simulink library "thermochemical"  (R2017b)
settings: Solver=VariableStepAuto  StartTime=0.0  StopTime=10.0  RelTol=1e-3
values from neighbouring files (symbols this model uses):
  c = conversion_factors()    [blk_clausius_clapeyron.m]    (also in blk_clausius_clapeyron_no_popup.m; blk_cold_room_closed_dry_air.m; blk_reactor_BaCl2_NH3_no_walls.m; blk_reactor_BaCl2_NH3_no_walls_state_space.m)
  cp = metal.cp    [blk_wall_simple.m]    (also in get_metal_properties.m = 390)
  fluid = get_param(blk,'fluid')    [blk_thermodynamic_properties_nonsaturated.m]    (also in blk_thermodynamic_properties_nonsaturated_interpreted.m; blk_thermodynamic_properties_saturated.m; blk_thermodynamic_properties_saturated_interpreted.m; blk_thermodynamic_properties_saturated_mix.m)
  gas = get_material_properties(x.gasName)    [blk_reactor_BaCl2_NH3_cylindrical_no_walls_fun1.m]
  h = get_param(gcb,'ObjectParameters')    [get_param_eval.m]
  rho = metal.rho    [blk_wall_simple.m]    (also in get_metal_properties.m = 8940)
  s = solve(eq,dx,'ReturnConditions',true)    [LMTD_inv.m]    (also in blk_wall_simple.m = get_param_eval(blk,'s'))
  u_gas_at_T_ref = -R * T_ref    [blk_reactor_BaCl2_NH3_no_walls.m]    (also in blk_reactor_BaCl2_NH3_no_walls_state_space.m)
undefined symbols (not defined in the file or in its folder): b_motor, BaCl2, beta, CoolProp, cP_binder, cP_gas, cP_s0, cv, dh_r_0, ENG, heat_exchanger_epsilonNTU_inv_simulink, heat_exchanger_epsilonNTU_simulink, J_motor, K_cin, kappa, Km_motor, La_motor, lookup2D_BreakPoint2, M_binder, N_binder, N_gas_free_volume_init, N_salt, NH3, nh3_v3, nu, P, phase, PID_D_motor, PID_I_motor, PID_P_motor, Ra_motor, Reactor_phase, T, T1, T2, T_init, Tr_init, Tr_ref, U_binder_at_Tr_ref, U_salt_at_X0_Tr_ref, Ur_init, V_void, Valve_regime, Vmax_motor, w_init_motor, X_init
libraries: thermochemical x247, simulink x54, dspsigops x3
(part 10 of 12)

== system thermochemical/Reactors/Reactor, BaCl2//NH3, with algebraic loops, real gas in void volume, ideal gas in salt/Reactor, BaCl2//NH3, no walls, with algebraic loops, real gas in void volume, ideal gas in salt/Reactor (no walls)/Reactor's temperature and pressure ==
  In2 : Inport
  In1 : Inport  Port=2
  "Reaction kinetic, differential equation" : Subsystem
  Reactor's energy balance : Subsystem
  Out3 : Outport
  Out1 : Outport  Port=2
  Out2 : Outport  Port=3
  Out4 : Outport  Port=4
  wires:
  "Reaction kinetic, differential equation"/1(Out1) -> Out2/1  "Reactor phase"
  Reactor's energy balance/2(Out2) -> Out1/1, "Reaction kinetic, differential equation"/2(In2)  "P_reactor (bar)"
  In2/1 -> Reactor's energy balance/2(In2)  "N_gas_reactor (mol)"
  Reactor's energy balance/1(Out1) -> Out3/1, "Reaction kinetic, differential equation"/1(In1)  "T_reactor (K)"
  "Reaction kinetic, differential equation"/2(Out2) -> Reactor's energy balance/3(In3), Out4/1  "X (0..1)"
  In1/1 -> Reactor's energy balance/1(In1)  "U_reactor (J)"

== system thermochemical/Reactors/Reactor, BaCl2//NH3, with algebraic loops, real gas in void volume, real gas in salt/Reactor, BaCl2//NH3, no walls, with algebraic loops, real gas in void volume, real gas in salt/Reactor (no walls)/Reactor's internal energy differential equation ==
  note: Reactor - Internal energy's
      | differential equation
  In1 : Inport
  In2 : Inport  Port=2
  In5 : Inport  Port=3
  In3 : Inport  Port=4
  1 : Constant  Value=X_init
  2 : Constant  Value=N_gas_free_volume_init
  3 : Constant  Value=Tr_init
  Integrator6 : Integrator  InitialConditionSource=external  InitialCondition=Ur_init
  Product4 : Product
  Reactor's internal energy equation : thermochemical/Reactors/Reactor's internal energy equation  Tr_ref=T_ref  N_salt=N_salt  cP_s0=cP_s0  U_salt_at_X0_Tr_ref=U_salt_at_X0_T_ref  N_binder=N_binder  M_binder=M_binder  cP_binder=cP_binder  U_binder_at_Tr_ref=U_binder_at_T_ref  V_void=V_void  gas_model_void_volume=Real gas model  gas_model_salt=Real gas model  is_ideal_gas_in_void_volume=-1  is_ideal_gas_in_salt=-1  fluid=fluid  cP_gas=cP_gas  u_gas_at_Tr_ref=u_gas_at_T_ref  nu=nu  dh_r=dh_r_0  R=8.314472
      settings: SourceProductName=@ Thermochemical
  Relay : Relay  OnSwitchValue=dn_dead_zone  OffSwitchValue=-dn_dead_zone  OffOutputValue=-1
  Sum19 : Sum  Inputs=++|
  Switch1 : Switch
  Out1 : Outport
  wires:
  In3/1 -> Relay/1, Product4/2  "dn_gas (mol/sec) > 0: gas in   < 0: gas out"
  In5/1 -> Switch1/3  "enthalpy out (J/mol)"
  In1/1 -> Sum19/1  "q out → in (W)"
  Sum19/1 -> Integrator6/1  "dUr"
  Integrator6/1 -> Out1/1  "U_reactor (J)"
  In2/1 -> Switch1/1  "enthalpy in (J/mol)"
  Switch1/1 -> Product4/1  "h_gas(Tgas)"
  Product4/1 -> Sum19/2  "dn_gas * h_gas"
  Reactor's internal energy equation/1 -> Integrator6/2
  1/1 -> Reactor's internal energy equation/1
  3/1 -> Reactor's internal energy equation/3
  2/1 -> Reactor's internal energy equation/2
  Relay/1 -> Switch1/2

== system thermochemical/Reactors/Reactor, BaCl2//NH3, with algebraic loops, real gas in void volume, real gas in salt/Reactor, BaCl2//NH3, no walls, with algebraic loops, real gas in void volume, real gas in salt/Reactor (no walls)/Reactor's temperature and pressure ==
  In2 : Inport
  In1 : Inport  Port=2
  "Reaction kinetic, differential equation" : Subsystem
  Reactor's energy balance : Subsystem
  Out3 : Outport
  Out1 : Outport  Port=2
  Out2 : Outport  Port=3
  Out4 : Outport  Port=4
  wires:
  In1/1 -> Reactor's energy balance/1(In1)  "U_reactor (J)"
  "Reaction kinetic, differential equation"/2(Out2) -> Out4/1, Reactor's energy balance/3(In3)  "X (0..1)"
  Reactor's energy balance/1(Out1) -> "Reaction kinetic, differential equation"/1(In1), Out3/1  "T_reactor (K)"
  In2/1 -> Reactor's energy balance/2(In2)  "N_gas_reactor (mol)"
  Reactor's energy balance/2(Out2) -> "Reaction kinetic, differential equation"/2(In2), Out1/1  "P_reactor (bar)"
  "Reaction kinetic, differential equation"/1(Out1) -> Out2/1  "Reactor phase"

== system thermochemical/Valves/Valve, liquid, IEC 60534-2-1:2012/Flow computation for incompressible fluids, IEC 60534-2-1:2012/dP sizing computation/dP chocked computation ==
  P upstream (bar)1 : Inport
  P upstream (bar)2 : Inport  Port=2
  P upstream (bar)3 : Inport  Port=3
  P upstream (bar)4 : Inport  Port=4
  Display1 : Display
  Display2 : Display
  Display3 : Display
  "Liquid critical pressure ratio factor, FF" : Subsystem
  Math Function : Math  Operator=square  SaturateOnIntegerOverflow=on
  Prod1 : Product  Inputs=**
  Prod2 : Product  Inputs=**
  Sum2 : Sum  Inputs=+-
  dP chocked (bar) : Outport
  wires:
  Sum2/1 -> Prod2/1
  Prod2/1 -> dP chocked (bar)/1  "dP chocked (bar)"
  Prod1/1 -> Display1/1, Sum2/2
  Math Function/1 -> Prod2/2
  P upstream (bar)4/1 -> Math Function/1  "FF factor"
  "Liquid critical pressure ratio factor, FF"/1(FF) -> Prod1/2, Display3/1
  P upstream (bar)3/1 -> "Liquid critical pressure ratio factor, FF"/2(P upstream (bar)1)  "Pc: absolute thermodynamic  critical pressure (bar)"
  P upstream (bar)1/1 -> Sum2/1  "P upstream (bar)"
  P upstream (bar)2/1 -> Prod1/1, Display2/1, "Liquid critical pressure ratio factor, FF"/1(P upstream (bar)2)  "Pv: absolute vapor pressure  of liquid at T upstream (bar)"

== system thermochemical/Walls/Wall, tube with//without fins/Subsystem1/Subsystem2/Subsystem1 ==
  In1 : Inport
  In2 : Inport  Port=2
  In3 : Inport  Port=3
  Gain1 : Gain  Gain=pi/4
  Gain2 : Gain  Gain=2
  Gain4 : Gain  Gain=1e-3
  Gain5 : Gain  Gain=1e-3
  Math Function : Math  Operator=square  SaturateOnIntegerOverflow=on
  Math Function1 : Math  Operator=square  SaturateOnIntegerOverflow=on
  Product2 : Product
  Sum1 : Sum  Inputs=+-
  Sum2 : Sum  Inputs=+-
  Inner area (m2) : Outport
  wires:
  Gain1/1 -> Product2/1
  Product2/1 -> Inner area (m2)/1  "Bare tube volume (m3)"
  In3/1 -> Product2/2  "L_m"
  In1/1 -> Gain4/1  "OD_mm"
  In2/1 -> Gain5/1  "e_mm"
  Sum1/1 -> Math Function1/1
  Math Function/1 -> Sum2/1
  Math Function1/1 -> Sum2/2
  Sum2/1 -> Gain1/1
  Gain4/1 -> Sum1/1, Math Function/1  "OD_m"
  Gain5/1 -> Gain2/1  "e_m"
  Gain2/1 -> Sum1/2

== system thermochemical/Walls/Wall, tube with//without fins/Subsystem1/Subsystem2/Subsystem2 ==
  In1 : Inport
  In2 : Inport  Port=2
  In4 : Inport  Port=3
  Gain1 : Gain  Gain=pi/4
  Gain3 : Gain  Gain=1e-3
  Gain4 : Gain  Gain=1e-3
  Gain5 : Gain  Gain=1e-3
  Math Function : Math  Operator=square  SaturateOnIntegerOverflow=on
  Math Function1 : Math  Operator=square  SaturateOnIntegerOverflow=on
  Product : Product
  Sum2 : Sum  Inputs=+-
  Sum3 : Sum
  Inner area (m2) : Outport
  wires:
  Product/1 -> Inner area (m2)/1  "Volume of  individual fin (m3)"
  Gain3/1 -> Product/2  "thickness_fin_m"
  In2/1 -> Gain3/1  "thickness_fin_mm"
  Sum3/1 -> Math Function/1
  Gain1/1 -> Product/1  "Individual one-side  area of fin (m2)"
  In1/1 -> Gain5/1  "OD_mm"
  In4/1 -> Gain4/1  "height_fin_mm"
  Math Function/1 -> Sum2/1
  Math Function1/1 -> Sum2/2
  Sum2/1 -> Gain1/1
  Gain4/1 -> Sum3/1  "height_fin_m"
  Gain5/1 -> Sum3/2, Math Function1/1  "OD_m"

== system thermochemical/Walls/Wall, tube with//without fins, with internal heat production/Subsystem1/Subsystem2/Subsystem1 ==
  In1 : Inport
  In2 : Inport  Port=2
  In3 : Inport  Port=3
  Gain1 : Gain  Gain=pi/4
  Gain2 : Gain  Gain=2
  Gain4 : Gain  Gain=1e-3
  Gain5 : Gain  Gain=1e-3
  Math Function : Math  Operator=square  SaturateOnIntegerOverflow=on
  Math Function1 : Math  Operator=square  SaturateOnIntegerOverflow=on
  Product2 : Product
  Sum1 : Sum  Inputs=+-
  Sum2 : Sum  Inputs=+-
  Inner area (m2) : Outport
  wires:
  Gain5/1 -> Gain2/1  "e_m"
  Gain4/1 -> Math Function/1, Sum1/1  "OD_m"
  Sum2/1 -> Gain1/1
  Math Function1/1 -> Sum2/2
  Math Function/1 -> Sum2/1
  Sum1/1 -> Math Function1/1
  In2/1 -> Gain5/1  "e_mm"
  In1/1 -> Gain4/1  "OD_mm"
  In3/1 -> Product2/2  "L_m"
  Product2/1 -> Inner area (m2)/1  "Bare tube volume (m3)"
  Gain1/1 -> Product2/1
  Gain2/1 -> Sum1/2

== system thermochemical/Walls/Wall, tube with//without fins, with internal heat production/Subsystem1/Subsystem2/Subsystem2 ==
  In1 : Inport
  In2 : Inport  Port=2
  In4 : Inport  Port=3
  Gain1 : Gain  Gain=pi/4
  Gain3 : Gain  Gain=1e-3
  Gain4 : Gain  Gain=1e-3
  Gain5 : Gain  Gain=1e-3
  Math Function : Math  Operator=square  SaturateOnIntegerOverflow=on
  Math Function1 : Math  Operator=square  SaturateOnIntegerOverflow=on
  Product : Product
  Sum2 : Sum  Inputs=+-
  Sum3 : Sum
  Inner area (m2) : Outport
  wires:
  Gain5/1 -> Math Function1/1, Sum3/2  "OD_m"
  Gain4/1 -> Sum3/1  "height_fin_m"
  Sum2/1 -> Gain1/1
  Math Function1/1 -> Sum2/2
  Math Function/1 -> Sum2/1
  In4/1 -> Gain4/1  "height_fin_mm"
  In1/1 -> Gain5/1  "OD_mm"
  Gain1/1 -> Product/1  "Individual one-side  area of fin (m2)"
  Sum3/1 -> Math Function/1
  In2/1 -> Gain3/1  "thickness_fin_mm"
  Gain3/1 -> Product/2  "thickness_fin_m"
  Product/1 -> Inner area (m2)/1  "Volume of  individual fin (m3)"

== system thermochemical/Reactors/Reactor, BaCl2//NH3, state-space form, [Tr, Ng, X] as state variables, no algebraic loops, ideal gas in void volume, ideal gas in salt/Reactor, BaCl2//NH3, no walls, state-space form, [Tr, Ng, X] as state variables, no algebraic loops, ideal gas in void volume/Reactor, no walls, state space form/Reactor output function/Reactor phase ==
  In1 : Inport
  3 : Constant  Value=P_dead_zone
  Abs : Abs
  Enumerated Constant : simulink/Sources/Enumerated Constant  OutDataTypeStr=Enum: Reactor_phase  Value=Reactor_phase.Synthesis  SampleTime=inf
      settings: SourceProductName=Simulink
  Enumerated Constant1 : simulink/Sources/Enumerated Constant  OutDataTypeStr=Enum: Reactor_phase  Value=Reactor_phase.Desorption  SampleTime=inf
      settings: SourceProductName=Simulink
  Enumerated Constant2 : simulink/Sources/Enumerated Constant  OutDataTypeStr=Enum: Reactor_phase  Value=Reactor_phase.No_reaction  SampleTime=inf
      settings: SourceProductName=Simulink
  Relay : Relay  OnSwitchValue=P_dead_zone  OffSwitchValue=-P_dead_zone  OffOutputValue=-1
  Sign : Signum
  Sum17 : Sum  Inputs=|+-
  Switch1 : Switch  Criteria=u2 > Threshold
  Switch2 : Switch  Criteria=u2 > Threshold
  Out1 : Outport
  wires:
  Switch2/1 -> Out1/1  "Reactor phase"
  Enumerated Constant/1 -> Switch1/1  "Synthesis"
  Enumerated Constant1/1 -> Switch1/3  "Decomposition (desporption)"
  Switch1/1 -> Switch2/1
  Enumerated Constant2/1 -> Switch2/3  "No reaction"
  In1/1 -> Relay/1, Abs/1  "ΔP"
  Relay/1 -> Switch1/2
  Sum17/1 -> Sign/1
  Abs/1 -> Sum17/1
  Sign/1 -> Switch2/2
  3/1 -> Sum17/2

== system thermochemical/Reactors/Reactor, BaCl2//NH3, state-space form, [Tr, Ng, X] as state variables, no algebraic loops, ideal gas in void volume, ideal gas in salt/Reactor, BaCl2//NH3, no walls, state-space form, [Tr, Ng, X] as state variables, no algebraic loops, ideal gas in void volume/Reactor, no walls, state space form/Reactor state-space functions/f1 ==
  In6 : Inport
  In1 : Inport  Port=2
  Demux : Demux  Outputs=3
  Demux1 : Demux  Outputs=3
  Enthalpy of ideal gas : thermochemical/Thermodynamic fluid properties/Enthalpy of ideal gas  T_ref=T_ref  cP_gas=cP_gas  h_gas_at_T_ref="u_gas_at_T_ref  + R * T_ref"
      settings: SourceProductName=@ Thermochemical
  Enthalpy of reaction per mole of gas : Constant  Value=dh_r_0  VectorParams1D=off
  Gain2 : Gain  Gain=nu*N_salt
  Internal energy of ideal gas : thermochemical/Thermodynamic fluid properties/Internal energy of ideal gas  T_ref=T_ref  Cv_gas=cV_gas  u_gas_at_T_ref=u_gas_at_T_ref
      settings: SourceProductName=@ Thermochemical
  Product : Product  Inputs=/*
  Product1 : Product
  Product4 : Product
  Reactor's internal energy differential equation : thermochemical/Reactors/Reactor, BaCl2//NH3, state-space form, [Ur, Ng, X] as state variables, no algebraic loops, ideal gas in void volume, ideal gas in salt/Reactor, BaCl2//NH3, no walls, state-space form, [Ur, Ng, X] as state variables, no algebraic loops, ideal gas in void volume, ideal gas in salt/Reactor, no walls, state space form/Reactor state-space functions/f1/Reactor's internal energy differential equation
      settings: SourceProductName=@ Thermochemical
  Sum : Sum  Inputs=-+
  Sum3 : Sum  Inputs=--+
  Sum4 : Sum  Inputs=+-
  denominator : Subsystem
  f3 : Subsystem
  Out2 : Outport
  wires:
  Enthalpy of reaction per mole of gas/1 -> Sum/1  "(J/mol of gas)"
  Sum/1 -> Sum4/1  "(J/mol gas)"
  Enthalpy of ideal gas/1 -> Sum/2, Reactor's internal energy differential equation/3  "h gas"
  Product1/1 -> Sum3/2  "(J/sec)"
  Product4/1 -> Sum3/1  "(J/sec)"
  Reactor's internal energy differential equation/1 -> Sum3/3  "(J/sec)"
  Sum3/1 -> Product/2  "(J/sec)"
  f3/1(Out2) -> Product4/1  "(1/sec)"
  Gain2/1 -> Product4/2  "(J)"
  Sum4/1 -> Gain2/1
  Internal energy of ideal gas/1 -> Product1/1, Sum4/2  "J/mol"
  denominator/1(Out2) -> Product/1  "J/K"
  Demux/1 -> f3/1(In6), Enthalpy of ideal gas/1, Internal energy of ideal gas/1, denominator/1(In6)  "x(1) = T (K)"
  Demux1/3 -> Reactor's internal energy differential equation/1  "u(3) = Q out→in (W)"
  In1/1 -> Demux1/1  "U"
  Demux1/1 -> Reactor's internal energy differential equation/4, Product1/2  "u(1) = dn/dt gas (mol/sec), > 0: gas in, < 0: gas out"
  Demux1/2 -> Reactor's internal energy differential equation/2  "u(2) = h gas in (J/mol)"
  Demux/3 -> f3/3(In2), denominator/3(In4)  "x(3) = X (0..1)"
  Demux/2 -> f3/2(In1), denominator/2(In3)  "x(2) = Ngas,total (mol)"
  Product/1 -> Out2/1  "dT/dt (K/sec)"
  In6/1 -> Demux/1  "X"

== system thermochemical/Reactors/Reactor, BaCl2//NH3, state-space form, [Tr, Ng, X] as state variables, no algebraic loops, ideal gas in void volume, ideal gas in salt/Reactor, BaCl2//NH3, no walls, state-space form, [Tr, Ng, X] as state variables, no algebraic loops, ideal gas in void volume/Reactor, no walls, state space form/Reactor state-space functions/f2 ==
  In6 : Inport
  In2 : Inport  Port=2
  Demux : Demux  Outputs=3
  Demux2 : Demux  Outputs=3
  Gain : Gain
  Terminator{,1..2,5..6} (5 alike) : Terminator
  Out2 : Outport
  wires:
  Demux/1 -> Terminator/1  "x(1) = T (K)"
  In6/1 -> Demux/1  "X"
  Gain/1 -> Out2/1  "dNgas,total/dt (mol/sec)"
  Demux/2 -> Terminator1/1  "x(2) = Ngas,total (mol)"
  Demux/3 -> Terminator2/1  "x(3) = X (0..1)"
  Demux2/3 -> Terminator5/1  "u(3) = Q out→in (W)"
  Demux2/1 -> Gain/1  "u(1) = dn/dt gas (mol/sec), > 0: gas in, < 0: gas out"
  Demux2/2 -> Terminator6/1  "u(2) = h gas in (J/mol)"
  In2/1 -> Demux2/1  "U"

== system thermochemical/Reactors/Reactor, BaCl2//NH3, state-space form, [Tr, Ng, X] as state variables, no algebraic loops, ideal gas in void volume, ideal gas in salt/Reactor, BaCl2//NH3, no walls, state-space form, [Tr, Ng, X] as state variables, no algebraic loops, ideal gas in void volume/Reactor, no walls, state space form/Reactor state-space functions/f3 ==
  In6 : Inport
  In2 : Inport  Port=2
  Demux : Demux  Outputs=3
  Demux2 : Demux  Outputs=3
  Terminator1 : Terminator
  Terminator5 : Terminator
  Terminator6 : Terminator
  f3 : Subsystem
  Out2 : Outport
  wires:
  In6/1 -> Demux/1  "X"
  Demux/3 -> f3/3(In2)  "x(3) = X (0..1)"
  Demux/2 -> f3/2(In1)  "x(2) = Ngas,total (mol)"
  Demux/1 -> f3/1(In6)  "x(1) = T (K)"
  f3/1(Out2) -> Out2/1  "dX/dt (1/sec)"
  In2/1 -> Demux2/1  "U"
  Demux2/1 -> Terminator1/1  "u(1) = dn/dt gas (mol/sec), > 0: gas in, < 0: gas out"
  Demux2/2 -> Terminator6/1  "u(2) = h gas in (J/mol)"
  Demux2/3 -> Terminator5/1  "u(3) = Q out→in (W)"

== system thermochemical/Reactors/Reactor, BaCl2//NH3, state-space form, [Tr, Ng, X] as state variables, no algebraic loops, real gas in void volume, ideal gas in salt/Reactor, BaCl2//NH3, no walls, state-space form, [Tr, Ng, X] as state variables, no algebraic loops, real gas in void volume, ideal gas in salt/Reactor, no walls, state space form/Reactor output function/Reactor phase ==
  In1 : Inport
  3 : Constant  Value=P_dead_zone
  Abs : Abs
  Enumerated Constant : simulink/Sources/Enumerated Constant  OutDataTypeStr=Enum: Reactor_phase  Value=Reactor_phase.Synthesis  SampleTime=inf
      settings: SourceProductName=Simulink
  Enumerated Constant1 : simulink/Sources/Enumerated Constant  OutDataTypeStr=Enum: Reactor_phase  Value=Reactor_phase.Desorption  SampleTime=inf
      settings: SourceProductName=Simulink
  Enumerated Constant2 : simulink/Sources/Enumerated Constant  OutDataTypeStr=Enum: Reactor_phase  Value=Reactor_phase.No_reaction  SampleTime=inf
      settings: SourceProductName=Simulink
  Relay : Relay  OnSwitchValue=P_dead_zone  OffSwitchValue=-P_dead_zone  OffOutputValue=-1
  Sign : Signum
  Sum17 : Sum  Inputs=|+-
  Switch1 : Switch  Criteria=u2 > Threshold
  Switch2 : Switch  Criteria=u2 > Threshold
  Out1 : Outport
  wires:
  3/1 -> Sum17/2
  Sign/1 -> Switch2/2
  Abs/1 -> Sum17/1
  Sum17/1 -> Sign/1
  Relay/1 -> Switch1/2
  In1/1 -> Abs/1, Relay/1  "ΔP"
  Enumerated Constant2/1 -> Switch2/3  "No reaction"
  Switch1/1 -> Switch2/1
  Enumerated Constant1/1 -> Switch1/3  "Decomposition (desporption)"
  Enumerated Constant/1 -> Switch1/1  "Synthesis"
  Switch2/1 -> Out1/1  "Reactor phase"

== system thermochemical/Reactors/Reactor, BaCl2//NH3, state-space form, [Tr, Ng, X] as state variables, no algebraic loops, real gas in void volume, ideal gas in salt/Reactor, BaCl2//NH3, no walls, state-space form, [Tr, Ng, X] as state variables, no algebraic loops, real gas in void volume, ideal gas in salt/Reactor, no walls, state space form/Reactor state-space functions/f1 ==
  In6 : Inport
  In1 : Inport  Port=2
  Demux : Demux  Outputs=3
  Demux1 : Demux  Outputs=3
  Enthalpy of ideal gas : thermochemical/Thermodynamic fluid properties/Enthalpy of ideal gas  T_ref=T_ref  cP_gas=cP_gas  h_gas_at_T_ref="u_gas_at_T_ref  + R * T_ref"
      settings: SourceProductName=@ Thermochemical
  Enthalpy of reaction per mole of gas : Constant  Value=dh_r_0  VectorParams1D=off
  Gain2 : Gain  Gain=nu*N_salt
  Product : Product  Inputs=/*
  Product1 : Product
  Product4 : Product
  Reactor's internal energy differential equation : thermochemical/Reactors/Reactor, BaCl2//NH3, state-space form, [Ur, Ng, X] as state variables, no algebraic loops, ideal gas in void volume, ideal gas in salt/Reactor, BaCl2//NH3, no walls, state-space form, [Ur, Ng, X] as state variables, no algebraic loops, ideal gas in void volume, ideal gas in salt/Reactor, no walls, state space form/Reactor state-space functions/f1/Reactor's internal energy differential equation
      settings: SourceProductName=@ Thermochemical
  Sum : Sum  Inputs=-+
  Sum3 : Sum  Inputs=--+
  Sum4 : Sum  Inputs=+-
  denominator : Subsystem
  f1 : Subsystem
  f2 : Subsystem
  f3 : Subsystem
  Out2 : Outport
  wires:
  In6/1 -> Demux/1  "X"
  Product/1 -> Out2/1  "dT/dt (K/sec)"
  Demux/2 -> denominator/2(In3), f1/2(In1), f2/2(In1), f3/2(In1)  "x(2) = Ngas,total (mol)"
  Demux/3 -> denominator/3(In4), f1/3(In2), f2/3(In2), f3/3(In2)  "x(3) = X (0..1)"
  Demux1/2 -> Reactor's internal energy differential equation/2  "u(2) = h gas in (J/mol)"
  Demux1/1 -> Product1/2, Reactor's internal energy differential equation/4  "u(1) = dn/dt gas (mol/sec), > 0: gas in, < 0: gas out"
  In1/1 -> Demux1/1  "U"
  Demux1/3 -> Reactor's internal energy differential equation/1  "u(3) = Q out→in (W)"
  Demux/1 -> denominator/1(In6), f1/1(In6), f2/1(In6), Enthalpy of ideal gas/1, f3/1(In6)  "x(1) = T (K)"
  f1/1(Out2) -> Reactor's internal energy differential equation/3
  denominator/1(Out2) -> Product/1  "J/K"
  f2/1(Out2) -> Product1/1, Sum4/2
  Sum/1 -> Sum4/1
  Sum4/1 -> Gain2/1
  Gain2/1 -> Product4/2  "(J)"
  f3/1(Out2) -> Product4/1  "(1/sec)"
  Sum3/1 -> Product/2  "(J/sec)"
  Reactor's internal energy differential equation/1 -> Sum3/3  "(J/sec)"
  Product4/1 -> Sum3/1  "(J/sec)"
  Product1/1 -> Sum3/2  "(J/sec)"
  Enthalpy of reaction per mole of gas/1 -> Sum/1  "(J/mol of gas)"
  Enthalpy of ideal gas/1 -> Sum/2  "h gas"

== system thermochemical/Reactors/Reactor, BaCl2//NH3, state-space form, [Tr, Ng, X] as state variables, no algebraic loops, real gas in void volume, ideal gas in salt/Reactor, BaCl2//NH3, no walls, state-space form, [Tr, Ng, X] as state variables, no algebraic loops, real gas in void volume, ideal gas in salt/Reactor, no walls, state space form/Reactor state-space functions/f2 ==
  In6 : Inport
  In2 : Inport  Port=2
  Demux : Demux  Outputs=3
  Demux2 : Demux  Outputs=3
  Gain : Gain
  Terminator{,1..2,5..6} (5 alike) : Terminator
  Out2 : Outport
  wires:
  In2/1 -> Demux2/1  "U"
  Demux2/2 -> Terminator6/1  "u(2) = h gas in (J/mol)"
  Demux2/1 -> Gain/1  "u(1) = dn/dt gas (mol/sec), > 0: gas in, < 0: gas out"
  Demux2/3 -> Terminator5/1  "u(3) = Q out→in (W)"
  Demux/3 -> Terminator2/1  "x(3) = X (0..1)"
  Demux/2 -> Terminator1/1  "x(2) = Ngas,total (mol)"
  Gain/1 -> Out2/1  "dNgas,total/dt (mol/sec)"
  In6/1 -> Demux/1  "X"
  Demux/1 -> Terminator/1  "x(1) = T (K)"

== system thermochemical/Reactors/Reactor, BaCl2//NH3, state-space form, [Tr, Ng, X] as state variables, no algebraic loops, real gas in void volume, ideal gas in salt/Reactor, BaCl2//NH3, no walls, state-space form, [Tr, Ng, X] as state variables, no algebraic loops, real gas in void volume, ideal gas in salt/Reactor, no walls, state space form/Reactor state-space functions/f3 ==
  In6 : Inport
  In2 : Inport  Port=2
  Demux : Demux  Outputs=3
  Demux2 : Demux  Outputs=3
  Terminator1 : Terminator
  Terminator5 : Terminator
  Terminator6 : Terminator
  f3 : thermochemical/Reactors/Reactor, BaCl2//NH3, state-space form, [Tr, Ng, X] as state variables, no algebraic loops, real gas in void volume, ideal gas in salt/Reactor, BaCl2//NH3, no walls, state-space form, [Tr, Ng, X] as state variables, no algebraic loops, real gas in void volume, ideal gas in salt/Reactor, no walls, state space form/Reactor state-space functions/f1/f3
      settings: SourceProductName=@ Thermochemical
  Out2 : Outport
  wires:
  Demux2/3 -> Terminator5/1  "u(3) = Q out→in (W)"
  Demux2/2 -> Terminator6/1  "u(2) = h gas in (J/mol)"
  Demux2/1 -> Terminator1/1  "u(1) = dn/dt gas (mol/sec), > 0: gas in, < 0: gas out"
  In2/1 -> Demux2/1  "U"
  f3/1 -> Out2/1  "dX/dt (1/sec)"
  Demux/1 -> f3/1  "x(1) = T (K)"
  Demux/2 -> f3/2  "x(2) = Ngas,total (mol)"
  Demux/3 -> f3/3  "x(3) = X (0..1)"
  In6/1 -> Demux/1  "X"

== system thermochemical/Reactors/Reactor, BaCl2//NH3, state-space form, [Tr, Ng, X] as state variables, no algebraic loops, real gas in void volume, real gas in salt/Reactor, BaCl2//NH3, no walls, state-space form, [Tr, Ng, X] as state variables, no algebraic loops, real gas in void volume, real gas in salt/Reactor, no walls, state space form/Reactor output function/Reactor phase ==
  In1 : Inport
  3 : Constant  Value=P_dead_zone
  Abs : Abs
  Enumerated Constant : simulink/Sources/Enumerated Constant  OutDataTypeStr=Enum: Reactor_phase  Value=Reactor_phase.Synthesis  SampleTime=inf
      settings: SourceProductName=Simulink
  Enumerated Constant1 : simulink/Sources/Enumerated Constant  OutDataTypeStr=Enum: Reactor_phase  Value=Reactor_phase.Desorption  SampleTime=inf
      settings: SourceProductName=Simulink
  Enumerated Constant2 : simulink/Sources/Enumerated Constant  OutDataTypeStr=Enum: Reactor_phase  Value=Reactor_phase.No_reaction  SampleTime=inf
      settings: SourceProductName=Simulink
  Relay : Relay  OnSwitchValue=P_dead_zone  OffSwitchValue=-P_dead_zone  OffOutputValue=-1
  Sign : Signum
  Sum17 : Sum  Inputs=|+-
  Switch1 : Switch  Criteria=u2 > Threshold
  Switch2 : Switch  Criteria=u2 > Threshold
  Out1 : Outport
  wires:
  Switch2/1 -> Out1/1  "Reactor phase"
  Enumerated Constant/1 -> Switch1/1  "Synthesis"
  Enumerated Constant1/1 -> Switch1/3  "Decomposition (desporption)"
  Switch1/1 -> Switch2/1
  Enumerated Constant2/1 -> Switch2/3  "No reaction"
  In1/1 -> Relay/1, Abs/1  "ΔP"
  Relay/1 -> Switch1/2
  Sum17/1 -> Sign/1
  Abs/1 -> Sum17/1
  Sign/1 -> Switch2/2
  3/1 -> Sum17/2

== system thermochemical/Reactors/Reactor, BaCl2//NH3, state-space form, [Tr, Ng, X] as state variables, no algebraic loops, real gas in void volume, real gas in salt/Reactor, BaCl2//NH3, no walls, state-space form, [Tr, Ng, X] as state variables, no algebraic loops, real gas in void volume, real gas in salt/Reactor, no walls, state space form/Reactor state-space functions/f1 ==
  In6 : Inport
  In1 : Inport  Port=2
  Demux : Demux  Outputs=3
  Demux1 : Demux  Outputs=3
  Gain2 : Gain  Gain=nu*N_salt
  Product : Product  Inputs=/*
  Product1 : Product
  Product4 : Product
  Reactor's internal energy differential equation : thermochemical/Reactors/Reactor, BaCl2//NH3, state-space form, [Ur, Ng, X] as state variables, no algebraic loops, ideal gas in void volume, ideal gas in salt/Reactor, BaCl2//NH3, no walls, state-space form, [Ur, Ng, X] as state variables, no algebraic loops, ideal gas in void volume, ideal gas in salt/Reactor, no walls, state space form/Reactor state-space functions/f1/Reactor's internal energy differential equation
      settings: SourceProductName=@ Thermochemical
  Sum3 : Sum  Inputs=--+
  Sum4 : Sum  Inputs=+-
  denominator : Subsystem
  f1 : Subsystem
  f2 : Subsystem
  f3 : Subsystem
  f4 : Subsystem
  Out2 : Outport
  wires:
  Product1/1 -> Sum3/2  "(J/sec)"
  Product4/1 -> Sum3/1  "(J/sec)"
  Reactor's internal energy differential equation/1 -> Sum3/3  "(J/sec)"
  Sum3/1 -> Product/2  "(J/sec)"
  f3/1(Out2) -> Product4/1  "(1/sec)"
  Gain2/1 -> Product4/2  "(J)"
  Sum4/1 -> Gain2/1
  f4/1(Out2) -> Sum4/1
  f2/1(Out2) -> Sum4/2, Product1/1
  denominator/1(Out2) -> Product/1  "J/K"
  f1/1(Out2) -> Reactor's internal energy differential equation/3
  Demux/1 -> f3/1(In6), f4/1(In6), f2/1(In6), f1/1(In6), denominator/1(In6)  "x(1) = T (K)"
  Demux1/3 -> Reactor's internal energy differential equation/1  "u(3) = Q out→in (W)"
  In1/1 -> Demux1/1  "U"
  Demux1/1 -> Reactor's internal energy differential equation/4, Product1/2  "u(1) = dn/dt gas (mol/sec), > 0: gas in, < 0: gas out"
  Demux1/2 -> Reactor's internal energy differential equation/2  "u(2) = h gas in (J/mol)"
  Demux/3 -> f3/3(In2), f2/3(In2), f1/3(In2), denominator/3(In4)  "x(3) = X (0..1)"
  Demux/2 -> f3/2(In1), f2/2(In1), f1/2(In1), denominator/2(In3)  "x(2) = Ngas,total (mol)"
  Product/1 -> Out2/1  "dT/dt (K/sec)"
  In6/1 -> Demux/1  "X"

== system thermochemical/Reactors/Reactor, BaCl2//NH3, state-space form, [Tr, Ng, X] as state variables, no algebraic loops, real gas in void volume, real gas in salt/Reactor, BaCl2//NH3, no walls, state-space form, [Tr, Ng, X] as state variables, no algebraic loops, real gas in void volume, real gas in salt/Reactor, no walls, state space form/Reactor state-space functions/f2 ==
  In6 : Inport
  In2 : Inport  Port=2
  Demux : Demux  Outputs=3
  Demux2 : Demux  Outputs=3
  Gain : Gain
  Terminator{,1..2,5..6} (5 alike) : Terminator
  Out2 : Outport
  wires:
  Demux/1 -> Terminator/1  "x(1) = T (K)"
  In6/1 -> Demux/1  "X"
  Gain/1 -> Out2/1  "dNgas,total/dt (mol/sec)"
  Demux/2 -> Terminator1/1  "x(2) = Ngas,total (mol)"
  Demux/3 -> Terminator2/1  "x(3) = X (0..1)"
  Demux2/3 -> Terminator5/1  "u(3) = Q out→in (W)"
  Demux2/1 -> Gain/1  "u(1) = dn/dt gas (mol/sec), > 0: gas in, < 0: gas out"
  Demux2/2 -> Terminator6/1  "u(2) = h gas in (J/mol)"
  In2/1 -> Demux2/1  "U"

== system thermochemical/Reactors/Reactor, BaCl2//NH3, state-space form, [Tr, Ng, X] as state variables, no algebraic loops, real gas in void volume, real gas in salt/Reactor, BaCl2//NH3, no walls, state-space form, [Tr, Ng, X] as state variables, no algebraic loops, real gas in void volume, real gas in salt/Reactor, no walls, state space form/Reactor state-space functions/f3 ==
  In6 : Inport
  In2 : Inport  Port=2
  Demux : Demux  Outputs=3
  Demux2 : Demux  Outputs=3
  Terminator1 : Terminator
  Terminator5 : Terminator
  Terminator6 : Terminator
  f3 : thermochemical/Reactors/Reactor, BaCl2//NH3, state-space form, [Tr, Ng, X] as state variables, no algebraic loops, real gas in void volume, real gas in salt/Reactor, BaCl2//NH3, no walls, state-space form, [Tr, Ng, X] as state variables, no algebraic loops, real gas in void volume, real gas in salt/Reactor, no walls, state space form/Reactor state-space functions/f1/f3
      settings: SourceProductName=@ Thermochemical
  Out2 : Outport
  wires:
  In6/1 -> Demux/1  "X"
  Demux/3 -> f3/3  "x(3) = X (0..1)"
  Demux/2 -> f3/2  "x(2) = Ngas,total (mol)"
  Demux/1 -> f3/1  "x(1) = T (K)"
  f3/1 -> Out2/1  "dX/dt (1/sec)"
  In2/1 -> Demux2/1  "U"
  Demux2/1 -> Terminator1/1  "u(1) = dn/dt gas (mol/sec), > 0: gas in, < 0: gas out"
  Demux2/2 -> Terminator6/1  "u(2) = h gas in (J/mol)"
  Demux2/3 -> Terminator5/1  "u(3) = Q out→in (W)"

== system thermochemical/Reactors/Reactor, BaCl2//NH3, state-space form, [Ur, Ng, X] as state variables, no algebraic loops, ideal gas in void volume, ideal gas in salt/Reactor, BaCl2//NH3, no walls, state-space form, [Ur, Ng, X] as state variables, no algebraic loops, ideal gas in void volume, ideal gas in salt/Reactor, no walls, state space form/Reactor output function/Reactor phase ==
  In1 : Inport
  3 : Constant  Value=P_dead_zone
  Abs : Abs
  Enumerated Constant : simulink/Sources/Enumerated Constant  OutDataTypeStr=Enum: Reactor_phase  Value=Reactor_phase.Synthesis  SampleTime=inf
      settings: SourceProductName=Simulink
  Enumerated Constant1 : simulink/Sources/Enumerated Constant  OutDataTypeStr=Enum: Reactor_phase  Value=Reactor_phase.Desorption  SampleTime=inf
      settings: SourceProductName=Simulink
  Enumerated Constant2 : simulink/Sources/Enumerated Constant  OutDataTypeStr=Enum: Reactor_phase  Value=Reactor_phase.No_reaction  SampleTime=inf
      settings: SourceProductName=Simulink
  Relay : Relay  OnSwitchValue=P_dead_zone  OffSwitchValue=-P_dead_zone  OffOutputValue=-1
  Sign : Signum
  Sum17 : Sum  Inputs=|+-
  Switch1 : Switch  Criteria=u2 > Threshold
  Switch2 : Switch  Criteria=u2 > Threshold
  Out1 : Outport
  wires:
  Switch2/1 -> Out1/1  "Reactor phase"
  Enumerated Constant/1 -> Switch1/1  "Synthesis"
  Enumerated Constant1/1 -> Switch1/3  "Decomposition (desporption)"
  Switch1/1 -> Switch2/1
  Enumerated Constant2/1 -> Switch2/3  "No reaction"
  In1/1 -> Relay/1, Abs/1  "ΔP"
  Relay/1 -> Switch1/2
  Sum17/1 -> Sign/1
  Abs/1 -> Sum17/1
  Sign/1 -> Switch2/2
  3/1 -> Sum17/2

== system thermochemical/Reactors/Reactor, BaCl2//NH3, state-space form, [Ur, Ng, X] as state variables, no algebraic loops, ideal gas in void volume, ideal gas in salt/Reactor, BaCl2//NH3, no walls, state-space form, [Ur, Ng, X] as state variables, no algebraic loops, ideal gas in void volume, ideal gas in salt/Reactor, no walls, state space form/Reactor state-space functions/f1 ==
  In6 : Inport
  In2 : Inport  Port=2
  Demux : Demux  Outputs=3
  Demux2 : Demux  Outputs=3
  Enthalpy of ideal gas : thermochemical/Thermodynamic fluid properties/Enthalpy of ideal gas  T_ref=T_ref  cP_gas=cP_gas  h_gas_at_T_ref="u_gas_at_T_ref  + R * T_ref"
      settings: SourceProductName=@ Thermochemical
  Reactor's internal energy differential equation : Subsystem
  Tr = inv(g[X(vector)]) : Subsystem
  Out2 : Outport
  wires:
  Demux2/3 -> Reactor's internal energy differential equation/1(In1)  "u(3) = Q out→in (W)"
  Demux2/2 -> Reactor's internal energy differential equation/2(In2)  "u(2) = h gas in (J/mol)"
  Demux2/1 -> Reactor's internal energy differential equation/4(In3)  "u(1) = dn/dt gas (mol/sec), > 0: gas in, < 0: gas out"
  In2/1 -> Demux2/1  "U (vector)"
  In6/1 -> Demux/1  "X (vector)"
  Reactor's internal energy differential equation/1(Out1) -> Out2/1  "dUr/dt (J/sec)"
  Demux/3 -> Tr = inv(g[X(vector)])/3(In4)  "x(3) = X (0..1)"
  Demux/1 -> Tr = inv(g[X(vector)])/1(In6)  "x(1) = Ur (J)"
  Demux/2 -> Tr = inv(g[X(vector)])/2(In3)  "x(2) = Ngas,total (mol)"
  Enthalpy of ideal gas/1 -> Reactor's internal energy differential equation/3(In5)
  Tr = inv(g[X(vector)])/1(Out2) -> Enthalpy of ideal gas/1

== system thermochemical/Reactors/Reactor, BaCl2//NH3, state-space form, [Ur, Ng, X] as state variables, no algebraic loops, ideal gas in void volume, ideal gas in salt/Reactor, BaCl2//NH3, no walls, state-space form, [Ur, Ng, X] as state variables, no algebraic loops, ideal gas in void volume, ideal gas in salt/Reactor, no walls, state space form/Reactor state-space functions/f2 ==
  In6 : Inport
  In2 : Inport  Port=2
  Demux : Demux  Outputs=3
  Demux2 : Demux  Outputs=3
  Gain : Gain
  Terminator{,1..2,5..6} (5 alike) : Terminator
  Out2 : Outport
  wires:
  Demux/1 -> Terminator/1  "x(1) = Ur (J)"
  In6/1 -> Demux/1  "X"
  Gain/1 -> Out2/1  "dNgas,total/dt (mol/sec)"
  Demux/2 -> Terminator1/1  "x(2) = Ngas,total (mol)"
  Demux/3 -> Terminator2/1  "x(3) = X (0..1)"
  Demux2/3 -> Terminator5/1  "u(3) = Q out→in (W)"
  Demux2/1 -> Gain/1  "u(1) = dn/dt gas (mol/sec), > 0: gas in, < 0: gas out"
  Demux2/2 -> Terminator6/1  "u(2) = h gas in (J/mol)"
  In2/1 -> Demux2/1  "U"

== system thermochemical/Reactors/Reactor, BaCl2//NH3, state-space form, [Ur, Ng, X] as state variables, no algebraic loops, ideal gas in void volume, ideal gas in salt/Reactor, BaCl2//NH3, no walls, state-space form, [Ur, Ng, X] as state variables, no algebraic loops, ideal gas in void volume, ideal gas in salt/Reactor, no walls, state space form/Reactor state-space functions/f3 ==
  In6 : Inport
  In2 : Inport  Port=2
  Demux : Demux  Outputs=3
  Demux2 : Demux  Outputs=3
  Terminator1 : Terminator
  Terminator5 : Terminator
  Terminator6 : Terminator
  Tr = inv(g[X(vector)]) : thermochemical/Reactors/Reactor, BaCl2//NH3, state-space form, [Ur, Ng, X] as state variables, no algebraic loops, ideal gas in void volume, ideal gas in salt/Reactor, BaCl2//NH3, no walls, state-space form, [Ur, Ng, X] as state variables, no algebraic loops, ideal gas in void volume, ideal gas in salt/Reactor, no walls, state space form/Reactor state-space functions/f1/Tr = inv(g[X(vector)])
      settings: SourceProductName=@ Thermochemical
  f3 : Subsystem
  Out2 : Outport
  wires:
  In6/1 -> Demux/1  "X"
  Demux/3 -> Tr = inv(g[X(vector)])/3, f3/3(In2)  "x(3) = X (0..1)"
  Demux/2 -> Tr = inv(g[X(vector)])/2, f3/2(In1)  "x(2) = Ngas,total (mol)"
  Demux/1 -> Tr = inv(g[X(vector)])/1  "x(1) = Ur (J)"
  f3/1(Out2) -> Out2/1  "dX/dt (1/sec)"
  In2/1 -> Demux2/1  "U"
  Demux2/1 -> Terminator1/1  "u(1) = dn/dt gas (mol/sec), > 0: gas in, < 0: gas out"
  Demux2/2 -> Terminator6/1  "u(2) = h gas in (J/mol)"
  Demux2/3 -> Terminator5/1  "u(3) = Q out→in (W)"
  Tr = inv(g[X(vector)])/1 -> f3/1(In6)

== system thermochemical/Reactors/Reactor, BaCl2//NH3, with algebraic loops, ideal gas in void volume, ideal gas in salt/Reactor, BaCl2//NH3, no walls, with algebraic loops, ideal gas in void volume, ideal gas in salt/Reactor (no walls)/Reactor's temperature and pressure/Reaction kinetic, differential equation ==
  note: Reaction's advancement
      | differential equation
  In1 : Inport
  In2 : Inport  Port=2
  Check Dynamic Range1 : simulink/Model Verification/Check  Dynamic Range  Description=min < u < max  enabled=on  stopWhenAssertionFail=on  export=off  icon=graphic
      settings: SourceProductName=Simulink  SourceProductBaseCode=SL
  Clausius-Clapeyron : thermochemical/Thermodynamic fluid properties/Clausius-Clapeyron  sel_1=P(T)  sel_2=BaCl2/NH3
      settings: SourceProductName=@ Thermochemical
  Integrator8 : Integrator  InitialCondition=X_init
  Mux : Mux  Inputs=3
  "Reaction kinetic, differential equation" : Subsystem
  Reactor phase : Subsystem
  Sum16 : Sum  Inputs=-+
  Terminator : Terminator
  Thermodynamic property (saturated) : thermochemical/Thermodynamic fluid properties/Thermodynamic  property (saturated)  sel=P(T) (bar)  fluid=fluid  lookup1D_BreakPoint1=fluid.sat.T  lookup1D_Data=fluid.sat.Psat
      settings: SourceProductName=@ Thermochemical
  dn_gas3 : Constant  Value=1+1e-5
  dn_gas5 : Constant  Value=-1e-5
  Out1 : Outport
  Out2 : Outport  Port=2
  wires:
  In2/1 -> Mux/1, Sum16/2, "Reaction kinetic, differential equation"/2(In2)  "P_reactor (bar)"
  "Reaction kinetic, differential equation"/1(Out2) -> Integrator8/1  "dX/dt (1/sec)"
  Integrator8/1 -> "Reaction kinetic, differential equation"/3(In3), Out2/1, Check Dynamic Range1/3  "X [0..1]"
  Clausius-Clapeyron/1 -> Sum16/1, Mux/2  "P_reactor_equilb (bar)"
  Sum16/1 -> Reactor phase/1(In1)  "dP"
  dn_gas3/1 -> Check Dynamic Range1/1
  dn_gas5/1 -> Check Dynamic Range1/2
  Mux/1 -> Terminator/1  "Pressures comparison"
  In1/1 -> Thermodynamic property (saturated)/1, Clausius-Clapeyron/1, "Reaction kinetic, differential equation"/1(In1)  "T_reactor (K)"
  Reactor phase/1(Out1) -> Out1/1  "Reactor phase"
  Thermodynamic property (saturated)/1 -> Mux/3  "P_sat_gas(T_reactor)"

== system thermochemical/Reactors/Reactor, BaCl2//NH3, with algebraic loops, ideal gas in void volume, ideal gas in salt/Reactor, BaCl2//NH3, no walls, with algebraic loops, ideal gas in void volume, ideal gas in salt/Reactor (no walls)/Reactor's temperature and pressure/Reactor's energy balance ==
  In1 : Inport
  In2 : Inport  Port=2
  In3 : Inport  Port=3
  Gain17 : Gain  Gain=nu * N_salt
  Sum2 : Sum  Inputs=|-+
  Temperature equation : Subsystem
  Void volume pressure equation (real model) : Subsystem
  Out1 : Outport
  Out2 : Outport  Port=2
  wires:
  Sum2/1 -> Temperature equation/3(In3), Void volume pressure equation (real model)/2(In1)  "N_gas_free_volume (mol)"
  Temperature equation/1(Out1) -> Void volume pressure equation (real model)/1(In2), Out1/1  "T_reactor (K)"
  In1/1 -> Temperature equation/1(In1)  "U_reactor (J)"
  In3/1 -> Temperature equation/2(In2), Gain17/1  "X ([0..1])"
  In2/1 -> Sum2/2  "N_gas_reactor (mol)"
  Gain17/1 -> Sum2/1  "N_gas_absorved"
  Void volume pressure equation (real model)/1(Out1) -> Out2/1  "P_reactor (bar)"

== system thermochemical/Reactors/Reactor, BaCl2//NH3, with algebraic loops, real gas in void volume, ideal gas in salt/Reactor, BaCl2//NH3, no walls, with algebraic loops, real gas in void volume, ideal gas in salt/Reactor (no walls)/Reactor's temperature and pressure/Reaction kinetic, differential equation ==
  note: Reaction's advancement
      | differential equation
  In1 : Inport
  In2 : Inport  Port=2
  Check Dynamic Range1 : simulink/Model Verification/Check  Dynamic Range  Description=min < u < max  enabled=on  stopWhenAssertionFail=on  export=off  icon=graphic
      settings: SourceProductName=Simulink  SourceProductBaseCode=SL
  Clausius-Clapeyron : thermochemical/Thermodynamic fluid properties/Clausius-Clapeyron  sel_1=P(T)  sel_2=BaCl2/NH3
      settings: SourceProductName=@ Thermochemical
  Integrator8 : Integrator  InitialCondition=X_init
  Mux : Mux  Inputs=3
  "Reaction kinetic, differential equation" : Subsystem
  Reactor phase : Subsystem
  Sum16 : Sum  Inputs=-+
  Terminator : Terminator
  Thermodynamic property (saturated) : thermochemical/Thermodynamic fluid properties/Thermodynamic  property (saturated)  sel=P(T) (bar)  fluid=fluid  lookup1D_BreakPoint1=fluid.sat.T  lookup1D_Data=fluid.sat.Psat
      settings: SourceProductName=@ Thermochemical
  dn_gas3 : Constant  Value=1+1e-5
  dn_gas5 : Constant  Value=-1e-5
  Out1 : Outport
  Out2 : Outport  Port=2
  wires:
  Thermodynamic property (saturated)/1 -> Mux/3  "P_sat_gas(T_reactor)"
  Reactor phase/1(Out1) -> Out1/1  "Reactor phase"
  In1/1 -> "Reaction kinetic, differential equation"/1(In1), Clausius-Clapeyron/1, Thermodynamic property (saturated)/1  "T_reactor (K)"
  Mux/1 -> Terminator/1  "Pressures comparison"
  dn_gas5/1 -> Check Dynamic Range1/2
  dn_gas3/1 -> Check Dynamic Range1/1
  Sum16/1 -> Reactor phase/1(In1)  "dP"
  Clausius-Clapeyron/1 -> Mux/2, Sum16/1  "P_reactor_equilb (bar)"
  Integrator8/1 -> Check Dynamic Range1/3, Out2/1, "Reaction kinetic, differential equation"/3(In3)  "X [0..1]"
  "Reaction kinetic, differential equation"/1(Out2) -> Integrator8/1  "dX/dt (1/sec)"
  In2/1 -> "Reaction kinetic, differential equation"/2(In2), Sum16/2, Mux/1  "P_reactor (bar)"

== system thermochemical/Reactors/Reactor, BaCl2//NH3, with algebraic loops, real gas in void volume, ideal gas in salt/Reactor, BaCl2//NH3, no walls, with algebraic loops, real gas in void volume, ideal gas in salt/Reactor (no walls)/Reactor's temperature and pressure/Reactor's energy balance ==
  In1 : Inport
  In2 : Inport  Port=2
  In3 : Inport  Port=3
  Gain17 : Gain  Gain=nu * N_salt
  Sum2 : Sum  Inputs=|-+
  Temperature equation : Subsystem
  Void volume pressure equation (real model) : Subsystem
  Out1 : Outport
  Out2 : Outport  Port=2
  wires:
  Void volume pressure equation (real model)/1(Out1) -> Out2/1  "P_reactor (bar)"
  Gain17/1 -> Sum2/1  "N_gas_absorved"
  In2/1 -> Sum2/2  "N_gas_reactor (mol)"
  In3/1 -> Gain17/1, Temperature equation/2(In2)  "X ([0..1])"
  In1/1 -> Temperature equation/1(In1)  "U_reactor (J)"
  Temperature equation/1(Out1) -> Out1/1, Void volume pressure equation (real model)/1(In2)  "T_reactor (K)"
  Sum2/1 -> Void volume pressure equation (real model)/2(In1), Temperature equation/3(In3)  "N_gas_free_volume (mol)"

== system thermochemical/Reactors/Reactor, BaCl2//NH3, with algebraic loops, real gas in void volume, real gas in salt/Reactor, BaCl2//NH3, no walls, with algebraic loops, real gas in void volume, real gas in salt/Reactor (no walls)/Reactor's temperature and pressure/Reaction kinetic, differential equation ==
  note: Reaction's advancement
      | differential equation
  In1 : Inport
  In2 : Inport  Port=2
  Check Dynamic Range1 : simulink/Model Verification/Check  Dynamic Range  Description=min < u < max  enabled=on  stopWhenAssertionFail=on  export=off  icon=graphic
      settings: SourceProductName=Simulink  SourceProductBaseCode=SL
  Clausius-Clapeyron : thermochemical/Thermodynamic fluid properties/Clausius-Clapeyron  sel_1=P(T)  sel_2=BaCl2/NH3
      settings: SourceProductName=@ Thermochemical
  Integrator8 : Integrator  InitialCondition=X_init
  Mux : Mux  Inputs=3
  "Reaction kinetic, differential equation" : Subsystem
  Reactor phase : Subsystem
  Sum16 : Sum  Inputs=-+
  Terminator : Terminator
  Thermodynamic property (saturated) : thermochemical/Thermodynamic fluid properties/Thermodynamic  property (saturated)  sel=P(T) (bar)  fluid=fluid  lookup1D_BreakPoint1=fluid.sat.T  lookup1D_Data=fluid.sat.Psat
      settings: SourceProductName=@ Thermochemical
  dn_gas3 : Constant  Value=1+1e-5
  dn_gas5 : Constant  Value=-1e-5
  Out1 : Outport
  Out2 : Outport  Port=2
  wires:
  In2/1 -> Mux/1, Sum16/2, "Reaction kinetic, differential equation"/2(In2)  "P_reactor (bar)"
  "Reaction kinetic, differential equation"/1(Out2) -> Integrator8/1  "dX/dt (1/sec)"
  Integrator8/1 -> "Reaction kinetic, differential equation"/3(In3), Out2/1, Check Dynamic Range1/3  "X [0..1]"
  Clausius-Clapeyron/1 -> Sum16/1, Mux/2  "P_reactor_equilb (bar)"
  Sum16/1 -> Reactor phase/1(In1)  "dP"
  dn_gas3/1 -> Check Dynamic Range1/1
  dn_gas5/1 -> Check Dynamic Range1/2
  Mux/1 -> Terminator/1  "Pressures comparison"
  In1/1 -> Thermodynamic property (saturated)/1, Clausius-Clapeyron/1, "Reaction kinetic, differential equation"/1(In1)  "T_reactor (K)"
  Reactor phase/1(Out1) -> Out1/1  "Reactor phase"
  Thermodynamic property (saturated)/1 -> Mux/3  "P_sat_gas(T_reactor)"

== system thermochemical/Reactors/Reactor, BaCl2//NH3, with algebraic loops, real gas in void volume, real gas in salt/Reactor, BaCl2//NH3, no walls, with algebraic loops, real gas in void volume, real gas in salt/Reactor (no walls)/Reactor's temperature and pressure/Reactor's energy balance ==
  In1 : Inport
  In2 : Inport  Port=2
  In3 : Inport  Port=3
  Gain17 : Gain  Gain=nu * N_salt
  Sum2 : Sum  Inputs=|-+
  Temperature equation : Subsystem
  Void volume pressure equation (real model) : Subsystem
  Out1 : Outport
  Out2 : Outport  Port=2
  wires:
  Sum2/1 -> Temperature equation/3(In3), Void volume pressure equation (real model)/2(In1)  "N_gas_free_volume (mol)"
  Temperature equation/1(Out1) -> Void volume pressure equation (real model)/1(In2), Out1/1  "T_reactor (K)"
  In1/1 -> Temperature equation/1(In1)  "U_reactor (J)"
  In3/1 -> Temperature equation/2(In2), Gain17/1  "X ([0..1])"
  In2/1 -> Sum2/2  "N_gas_reactor (mol)"
  Gain17/1 -> Sum2/1  "N_gas_absorved"
  Void volume pressure equation (real model)/1(Out1) -> Out2/1  "P_reactor (bar)"

== system thermochemical/Valves/Valve, liquid, IEC 60534-2-1:2012/Flow computation for incompressible fluids, IEC 60534-2-1:2012/dP sizing computation/dP chocked computation/Liquid critical pressure ratio factor, FF ==
  P upstream (bar)2 : Inport
  P upstream (bar)1 : Inport  Port=2
  Constant : Constant  Value=0.96
  Display3 : Display
  Divide1 : Product  Inputs=*/
  Gain3 : Gain  Gain=0.28
  Sqrt : Sqrt  SaturateOnIntegerOverflow=on
  Sum1 : Sum  Inputs=+-
  FF : Outport
  wires:
  Constant/1 -> Sum1/1
  Sqrt/1 -> Gain3/1
  Gain3/1 -> Display3/1, Sum1/2
  Sum1/1 -> FF/1  "FF"
  Divide1/1 -> Sqrt/1
  P upstream (bar)1/1 -> Divide1/2  "Pc: absolute thermodynamic  critical pressure (bar)"
  P upstream (bar)2/1 -> Divide1/1  "Pv: absolute vapor pressure  of liquid at T upstream (bar)"

== system thermochemical/Reactors/Reactor, BaCl2//NH3, state-space form, [Tr, Ng, X] as state variables, no algebraic loops, ideal gas in void volume, ideal gas in salt/Reactor, BaCl2//NH3, no walls, state-space form, [Tr, Ng, X] as state variables, no algebraic loops, ideal gas in void volume/Reactor, no walls, state space form/Reactor state-space functions/f1/denominator ==
  In6 : Inport
  In3 : Inport  Port=2
  In4 : Inport  Port=3
  Gain1 : Gain  Gain=cV_gas
  Gain2 : Gain  Gain=cP_gas
  Gain4 : Gain  Gain=nu*N_salt
  K1 : Constant  Value=N_salt*cP_s0 + N_binder*M_binder*cP_binder  VectorParams1D=off
  Sum : Sum  Inputs=3
  Sum5 : Sum  Inputs=|+-
  Terminator : Terminator
  Out2 : Outport
  wires:
  In6/1 -> Terminator/1  "T (K)"
  Gain2/1 -> Sum/3  "(J/K)"
  Gain4/1 -> Gain2/1, Sum5/2  "(mol gas/mol salt * mol salt = mol gas)"
  Gain1/1 -> Sum/2  "(J/K)"
  In3/1 -> Sum5/1  "Ngas,total (mol)"
  In4/1 -> Gain4/1  "X (0..1)"
  Sum5/1 -> Gain1/1  "Ngas,void"
  Sum/1 -> Out2/1  "denominator (J/K)"
  K1/1 -> Sum/1  "(J/K)"

== system thermochemical/Reactors/Reactor, BaCl2//NH3, state-space form, [Tr, Ng, X] as state variables, no algebraic loops, ideal gas in void volume, ideal gas in salt/Reactor, BaCl2//NH3, no walls, state-space form, [Tr, Ng, X] as state variables, no algebraic loops, ideal gas in void volume/Reactor, no walls, state space form/Reactor state-space functions/f1/f3 ==
  In6 : Inport
  In1 : Inport  Port=2
  In2 : Inport  Port=3
  Gain4 : Gain  Gain=nu*N_salt
  Gain7 : Gain  Gain=1/V_void
  Ideal gas equation of state : thermochemical/Thermodynamic fluid properties/Ideal gas equation of state  sel=P(T,rho)  R=8.3145  Pa_to_bar=1e-5  bar_to_Pa=1e5
      settings: SourceProductName=@ Thermochemical
  "Reaction kinetic, differential equation" : Subsystem
  Sum2 : Sum  Inputs=|+-
  Out2 : Outport
  wires:
  "Reaction kinetic, differential equation"/1(Out2) -> Out2/1  "dX/dt (1/sec)"
  Ideal gas equation of state/1 -> "Reaction kinetic, differential equation"/2(In2)
  Sum2/1 -> Gain7/1  "Ngas,void"
  Gain7/1 -> Ideal gas equation of state/2
  Gain4/1 -> Sum2/2
  In6/1 -> "Reaction kinetic, differential equation"/1(In1), Ideal gas equation of state/1  "T (K)"
  In1/1 -> Sum2/1  "Ngas,total (mol)"
  In2/1 -> Gain4/1, "Reaction kinetic, differential equation"/3(In3)  "X (0..1)"
